simulink model "OpenLoopLinear"  (R2018a)
settings: Solver=VariableStepAuto  StartTime=0.0  StopTime=10.0  RelTol=1e-6
settings Model: Creator=melab2  LastModifiedBy=rahul

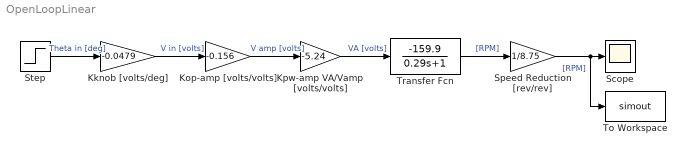
== system OpenLoopLinear ==
  Kknob [volts/deg] : Gain  Gain=-0.0479
  Kop-amp [volts/volts] : Gain  Gain=-0.156
  Kpw-amp VA/Vamp [volts/volts] : Gain  Gain=-5.24
  Scope : Scope
  Speed Reduction [rev/rev] : Gain  Gain=1/8.75
  Step : Step  After=120  SampleTime=0
  To Workspace : ToWorkspace  VariableName=simout  SampleTime=-1
  "Transfer Fcn " : TransferFcn  Numerator=-159.9  Denominator=[0.29 1]
  wires:
  Kpw-amp VA/Vamp [volts/volts]/1 -> "Transfer Fcn "/1  "VA [volts]"
  Kop-amp [volts/volts]/1 -> Kpw-amp VA/Vamp [volts/volts]/1  "V amp [volts]"
  Kknob [volts/deg]/1 -> Kop-amp [volts/volts]/1  "V in [volts]"
  Step/1 -> Kknob [volts/deg]/1  "Theta in [deg]"
  "Transfer Fcn "/1 -> Speed Reduction [rev/rev]/1  "[RPM]"
  Speed Reduction [rev/rev]/1 -> To Workspace/1, Scope/1  "[RPM]"
